simulink model "Prescan_Carsim_0118_repair_cs"  (R2019b)
settings: Solver=ode5  StartTime=0.0  StopTime=inf  FixedStep=1/1000  RelTol=1e-3
PreLoadFcn:
  | mbxruntime.callbacks.PreLoadFcn(bdroot);
PostLoadFcn:
  | mbxruntime.callbacks.PostLoadFcn(bdroot);
InitFcn:
  | mbxruntime.callbacks.InitFcn(bdroot);
  | Initialization_Func;
  | %T01_Init_2106;
StartFcn:
  | mbxruntime.callbacks.StartFcn(bdroot);
  | current_sys=gcs;
  | speedblock=Simulink.findBlocks(current_sys,'Name','speed_kmh_Gain');
  | h1=add_exec_event_listener(speedblock,'PostOutputs',@SpeedVisulization);
  | outblock=Simulink.findBlocks(current_sys,'Name','trajectorycurveoutput_Gain');
  | CurveTrajectoryListenerHandle=add_exec_event_listener(outblock,'PostOutputs',@TrajectoryCurve_CallBack);
  | lanedatablock=Simulink.findBlocks(current_sys,'Name','LaneData_Gain');
  | CurveLaneListenerHandle=add_exec_event_listener(lanedatablock,'PostOutputs',@CurveLane_CallBack);
StopFcn:
  | mbxruntime.callbacks.StopFcn(bdroot);
model workspace: external: MAT-File .\Prescan_Carsim_1230_cs_hws.mat (data not in the file)
undefined symbols (not defined in the file or in its folder): AAx, AAy, AAz, AVx, AVy, AVz, Ax, Ay, Az, canChannel, DiscIntNeverNeededParam, g, InitialDPMPDF_Comfort, InitialDPMPDF_Efficiency, InitialDPMPDF_Safety, InitialPDF_DEM, InitialPlanningParameter, Kf, Kr, Lr, M, mbxruntime, nG, NormalisedTrajectoryIndicator_Pool, Parameter_Indicator_LookUpTable, Prescan_Carsim_1230_cs_0658e9ca1334a8be, Prescan_Carsim_1230_cs_08c5eb9a1bd7376a, Prescan_Carsim_1230_cs_6cfd759b89b9fc85, Prescan_Carsim_1230_cs_9435cc1cceb5050d, Prescan_Carsim_1230_cs_ac716d34d49f74ab, Prescan_Carsim_1230_cs_be02757d7f212dd5, Rational_Coefficient_Learning, SteeringWheel, TrajectoryIndicatorRange, V, VehicleBaseLength, Vx, Vy, Vz, WheelL0, WheelL1, WheelR0, WheelR1
libraries: canmsglib x11, dsparch4 x6, canlib x3, PreScanSimulinkLibrary x3, Solver_SF x1, autolibshared x1
(part 1 of 8)
CloseFcn:
  | mbxruntime.callbacks.CloseFcn(bdroot);
settings Model: NumberOfSteps=100  Creator=PRESCAN  LastModifiedBy=CECLAB
settings DataIOCC: LimitDataPoints=on  SaveFormat=Array  SignalLoggingSaveFormat=ModelDataLogs  ReturnWorkspaceOutputs=off
settings OptimizationCC: DefaultParameterBehavior=Inlined  OptimizeBlockIOStorage=off  BufferReuse=off  GlobalBufferReuse=off  ExpressionFolding=off  ExpressionDepthLimit=2147483647  LocalBlockOutputs=off  InitFltsAndDblsToZero=on  LifeSpan=inf  OptimizeDataStoreBuffers=off  BusAssignmentInplaceUpdate=off
settings DebuggingCC: SaveWithParameterizedLinksMsg=none  UnderspecifiedInitializationDetection=Classic  MergeDetectMultiDrivingBlocksExec=none  SignalResolutionControl=TryResolveAllWithWarning  MultiTaskDSMMsg=warning  MultiTaskCondExecSysMsg=none  FcnCallInpInsideContextMsg=warning  StateNameClashWarn=warning  SFUnexpectedBacktrackingDiag=warning  SFNoUnconditionalDefaultTransitionDiag=warning  SFExecutionAtInitializationDiag=none  ArithmeticOperatorsInVariantConditions=warning
settings HardwareCC: ProdBitPerPointer=32  ProdBitPerSizeT=32  ProdBitPerPtrDiffT=32  ProdLargestAtomicFloat=None  ProdIntDivRoundTo=Undefined  ProdEndianess=Unspecified  ProdWordSize=32  ProdHWDeviceType=32-bit Generic
settings ModelReferenceCC: UpdateModelReferenceTargets=IfOutOfDate  PropagateSignalLabelsOutOfModel=off
settings SFSimCC: SimUseLocalCustomCode=off  SimParseCustomCode=off  CustomCodeUndefinedFunction=UseInterfaceOnly
settings SFSimCC: SimCustomHeaderCode=|
  | #include "prescan_alms_data.h"
  | #include "prescan.h"
  | #include "prescan_platform.h"
  | #include "prescan_aimsunturnindicatorsetter_data.h"
settings RTWCC: RTWUseLocalCustomCode=off
settings CodeAppCC: StateflowObjectComments=on
settings GRTTargetCC: TargetFcnLib=ansi_tfl_tmw.mat  TargetLangStandard=C89/C90 (ANSI)  GeneratePreprocessorConditionals=Disable all  CombineOutputUpdateFcns=off  GRTInterface=on
settings ConfigComp: CovMetricSettings=dw  CovHtmlReporting=on  CovSaveCumulativeToWorkspaceVar=on  CovSaveSingleToWorkspaceVar=on  CovExternalEMLEnable=off  CovSFcnEnable=off

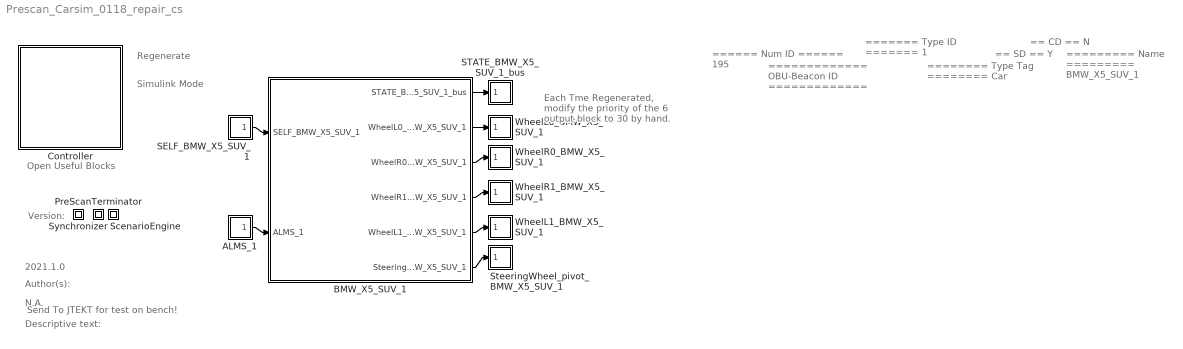
== system Prescan_Carsim_0118_repair_cs ==
  note: Each Tme Regenerated, modify the priority of the 6 output block to 30 by hand.
  note: Regenerate
  note: Simulink Mode
  note: Open Useful Blocks
  note: 2021.1.0
  note: Version:
  note: Author(s):
  note: N.A.
  note: Descriptive text:
  note: Send To JTEKT for test on bench!
  note: ======
      | Num ID
      | ======
      | 195
  note: =============
      | OBU-Beacon ID
      | =============
  note: =======
      | Type ID
      | =======
      | 1
  note: ========
      | Type Tag
      | ========
      | Car
  note: ==
      | SD
      | ==
      | Y
  note: ==
      | CD
      | ==
      | N
  note: =========
      | Name
      | =========
      | BMW_X5_SUV_1
  ALMS_1 : Subsystem  Tag=sensor/ALMS  Priority=30  LoadFcn=load('PrescanALMSData.mat');load('PrescanALMSMessage.mat');load('PrescanALMSPolynomial.mat')  mask(Analytical Lane Marker Sensor (ALMS) I/O){}
      mask help: The Analytical Lane Marker Sensor (ALMS) is a implementation of the Lane Marker Sensor, which provides information about the lane lines on the roads which are in view of the sensor.
      settings: OpenFcn=open_system([gcb '/Sensor'],'mask')
      mask Help: eval('openHelp(1466)')
      mask Display: image(imread('LaneMarkerSensorSL.png'))
  BMW_X5_SUV_1 : Subsystem  Tag=WorldObjectSubSystem  InitFcn=UniqueId = '1798';
      mask init:
      | modelPath = GenericModelHelper.getGenericModelFilePath('ModelDepo','Vehicles\BMW_X5\BMW_X5.pgmb','bfeb1c11467705ab888b3011684c848b');imagePath = GenericModelHelper.getCompilationPicture(modelPath, 'BMW_X5_HighPoly.png');
      mask Display: image(imread(imagePath));color('white');text(0, 0, ' ID=195\n')
  Controller : Subsystem  Description=8A3CD2955739A82C886C20AE3E253D78460D53180EE2C1B14CC08DF75A70BE77  Priority=-1  LoadFcn=load PreScanControllerData  mask(PreScan Simulation Controller){prescanversion='2021.1.0', ModelReferencing=off, TimeStep=50/1000, ControlMode=0, PreScanExecutionMode=on, ControllerCount=0, ControllerIndex=0, ControllerOptions=''}
      mask prompts: prescanversion "PreScan Version"; ModelReferencing "Use Model Referencing"; TimeStep "Upload Period [s]"; ControlMode "Control Mode"; PreScanExecutionMode "Execution Mode"; ControllerCount "Controller Count"; ControllerIndex "Controller Index"; ControllerOptions "Controller Options"
      mask help:
      | Please do not remove this block from the compilation sheet,
      | as it connects the model to the PreScan environment.
      mask init:
      | model = bdroot(gcb);
      | ExperimentFile = mbxruntime.findExperimentFile(model,true); %relative path
      | 
      | [d1, d2, d3, prescandata] = prescan_Settings();
      | ModelDepo = fullfile(prescandata,'ModelDepo'); 
      | 
      | RTmode = mbxruntime.getRTMode(model);
      | 
      | SimulationMode = get_param(bdroot,'SimulationMode');
      | if strcmp(SimulationMode, 'rapid-accelerator')
      |     SimulationMode = 'external';
      | end
      | TargetName = get_param(bdroot,'SystemTargetFile');
      settings: ModelCloseFcn=assignin('base',['model_closed_' bdroot],true);
      mask Help: eval('openHelp(812)')
      mask Display: image(imread('prescanlogo.ico'))
  PreScanTerminator : Subsystem  Tag=PreScanTerminator  Priority=999  LoadFcn=load PrescanTerminatorData  mask(PreScan Simulation Terminator){TimeStep=50/1000}
      mask prompts: TimeStep "Upload Period [s]"
      mask help:
      | Please do not remove this block from the compilation sheet as it
      | connects the model to the PreScan environment.
      mask Help: eval('openHelp(812)')
      mask Display: image(imread('prescanlogo.ico'))
  SELF_BMW_X5_SUV_1 : Subsystem  Tag=sensor/SelfPort  Priority=30  LoadFcn=load('PreScanSelfSensorData.mat')  mask(PreScan Source Block: SELF){}
      mask help:
      | The SELF port shows (state) information of the actor itself. The outputs are position in the experiment's axis system and the GPS coordinates, and the object's absolute velocity and compass heading.
      |
      | For more information, please click Help.
      settings: OpenFcn=open_system([gcb '/Sensor'],'mask')
      mask Help: eval('openHelp(462)')
      mask Display: image(imread('GPS.png'))
  STATE_BMW_X5_SUV_1_bus : Subsystem  Tag=actuator/StatePort  Priority=30  LoadFcn=load('PreScanStateActuatorData.mat')  mask(PreScan Sink Block: State){}
      mask help:
      | The Actor State contains a vector signal of size (9x1), containing the following signals:
      |
      | -  Position    	(x,y,z)             	[m]
      | -  Velocity    	(vx,vy,vz)         	[m/s]
      | -  Angles       	(Roll, Pitch, Yaw)	[rad]
      |
      | The Actor state is defined in the global axis system.
      | The state is superponed on the Initial position defined in the GUI.
      |
      | For more information, please click Help.
      settings: OpenFcn=open_system([gcb '/Actuator'],'mask')
      mask Help: eval('openHelp(222)')
      mask Display: image(imread('State.png'))
  ScenarioEngine : Subsystem  Tag=PreScanOpenScenarioBlock  Priority=0  LoadFcn=load PrescanSynchronizeData  mask(PreScan Simulation Core Block){TimeStep=50/1000}
      mask prompts: TimeStep "Timestep [s]"
      mask help:
      | Please do not remove this block from the PreScan compilation sheet,
      | as it contains essential configuration parameters for a PreScan simulation.
      settings: DeleteFcn=PreScanBlockDeleteFcn;
      mask Display: image(imread('prescanlogo.ico'))
  SteeringWheel_pivot_BMW_X5_SUV_1 : Subsystem  Tag=Actuator  Priority=30  LoadFcn=load('PrescanPoseData');load('PrescanXYZData');load('PreScanRPYData')
      mask help:
      | The VisuJoint block provides a way to adapt the location and orientation of a part of an object.
      |
      | For more information, please click Help.
      settings: OpenFcn=open_system([gcb '/Actuator'],'mask')
      mask Display: image(imread('Joint.png'))
  Synchronizer : Subsystem  Tag=PreScanSynchronizer  Priority=0  LoadFcn=load PrescanSynchronizeData  mask(PreScan Simulation Core Block){TimeStep=50/1000}
      mask prompts: TimeStep "Timestep [s]"
      mask help:
      | Please do not remove this block from the PreScan compilation sheet,
      | as it contains essential configuration parameters for a PreScan simulation.
      settings: DeleteFcn=PreScanBlockDeleteFcn;
      mask Display: image(imread('prescanlogo.ico'))
  WheelL0_BMW_X5_SUV_1 : Subsystem  Tag=Actuator  Priority=30  LoadFcn=load('PrescanPoseData');load('PrescanXYZData');load('PreScanRPYData')
      mask help:
      | The VisuJoint block provides a way to adapt the location and orientation of a part of an object.
      |
      | For more information, please click Help.
      settings: OpenFcn=open_system([gcb '/Actuator'],'mask')
      mask Display: image(imread('Joint.png'))
  WheelL1_BMW_X5_SUV_1 : Subsystem  Tag=Actuator  Priority=30  LoadFcn=load('PrescanPoseData');load('PrescanXYZData');load('PreScanRPYData')
      mask help:
      | The VisuJoint block provides a way to adapt the location and orientation of a part of an object.
      |
      | For more information, please click Help.
      settings: OpenFcn=open_system([gcb '/Actuator'],'mask')
      mask Display: image(imread('Joint.png'))
  WheelR0_BMW_X5_SUV_1 : Subsystem  Tag=Actuator  Priority=30  LoadFcn=load('PrescanPoseData');load('PrescanXYZData');load('PreScanRPYData')
      mask help:
      | The VisuJoint block provides a way to adapt the location and orientation of a part of an object.
      |
      | For more information, please click Help.
      settings: OpenFcn=open_system([gcb '/Actuator'],'mask')
      mask Display: image(imread('Joint.png'))
  WheelR1_BMW_X5_SUV_1 : Subsystem  Tag=Actuator  Priority=30  LoadFcn=load('PrescanPoseData');load('PrescanXYZData');load('PreScanRPYData')
      mask help:
      | The VisuJoint block provides a way to adapt the location and orientation of a part of an object.
      |
      | For more information, please click Help.
      settings: OpenFcn=open_system([gcb '/Actuator'],'mask')
      mask Display: image(imread('Joint.png'))
  wires:
  SELF_BMW_X5_SUV_1/1(SELF_BMW_X5_SUV_1) -> BMW_X5_SUV_1/1(SELF_BMW_X5_SUV_1)
  BMW_X5_SUV_1/1(STATE_BMW_X5_SUV_1_bus) -> STATE_BMW_X5_SUV_1_bus/1(STATE_BMW_X5_SUV_1_bus)
  ALMS_1/1(ALMS_1) -> BMW_X5_SUV_1/2(ALMS_1)
  BMW_X5_SUV_1/2(WheelL0_BMW_X5_SUV_1) -> WheelL0_BMW_X5_SUV_1/1(WheelL0_BMW_X5_SUV_1)
  BMW_X5_SUV_1/3(WheelR0_BMW_X5_SUV_1) -> WheelR0_BMW_X5_SUV_1/1(WheelR0_BMW_X5_SUV_1)
  BMW_X5_SUV_1/4(WheelR1_BMW_X5_SUV_1) -> WheelR1_BMW_X5_SUV_1/1(WheelR1_BMW_X5_SUV_1)
  BMW_X5_SUV_1/5(WheelL1_BMW_X5_SUV_1) -> WheelL1_BMW_X5_SUV_1/1(WheelL1_BMW_X5_SUV_1)
  BMW_X5_SUV_1/6(SteeringWheel_pivot_BMW_X5_SUV_1) -> SteeringWheel_pivot_BMW_X5_SUV_1/1(SteeringWheel_pivot_BMW_X5_SUV_1)

== system Prescan_Carsim_0118_repair_cs/ALMS_1 ==
  Sensor : S-Function  FunctionName=sfun_ALMS  Parameters=mbxruntime.parameters.convert(sensorID), mbxruntime.parameters.convert(detectableObjects), mbxruntime.parameters.convert(timestep)  SFunctionDeploymentMode=off  EnableBusSupport=off  mask(Analytical Lane Marker Sensor (ALMS) I/O){sensorID=15468, detectableObjects=30, timestep=1/20}
      mask prompts: sensorID "Sensor ID"; detectableObjects "Max detectable objects:"; timestep "MATLAB timestep:"
      mask help: The Analytical Lane Marker Sensor (ALMS) is a implementation of the Lane Marker Sensor, which provides information about the lane lines on the roads which are in view of the sensor.
      mask Help: eval('openHelp(1466)')
      mask Display: image(imread('LaneMarkerSensorSL.png'))
  ALMS_1 : Outport  Tag=outport/ALMS  OutDataTypeStr=Bus: PRESCAN_ALMS_MESSAGE  PortDimensions=30  SampleTime=1/20
  wires:
  Sensor/1 -> ALMS_1/1

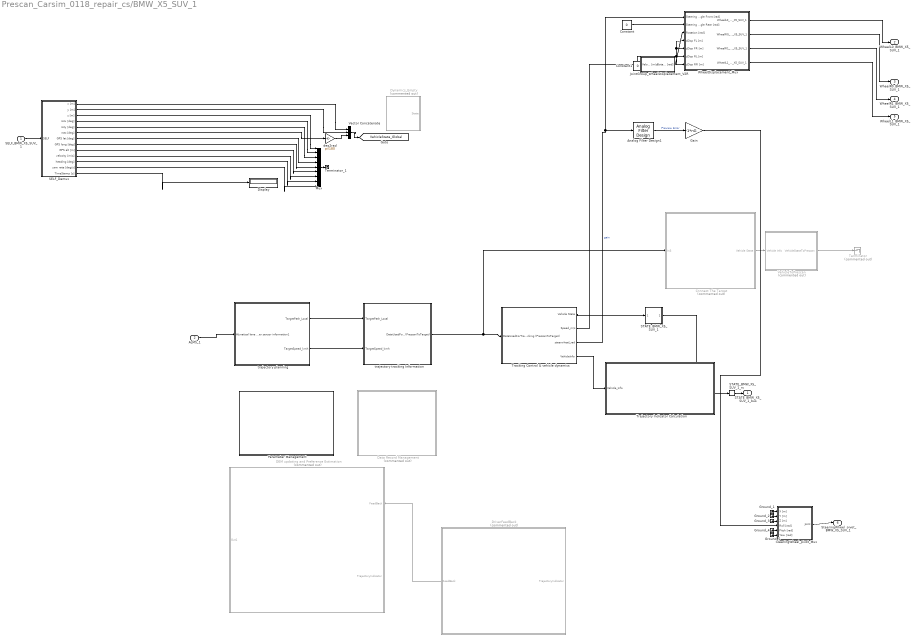
== system Prescan_Carsim_0118_repair_cs/BMW_X5_SUV_1 ==
  SELF_BMW_X5_SUV_1 : Inport  Tag=inport/SelfPort  OutDataTypeStr=Bus: PRESCAN_SELFSENSORDATA  PortDimensions=1  SampleTime=50/1000  BusOutputAsStruct=on
  ALMS_1 : Inport  Tag=inport/ALMS  Port=2  OutDataTypeStr=Bus: PRESCAN_ALMS_MESSAGE  PortDimensions=30  SampleTime=1/20  BusOutputAsStruct=on
  Analog Filter Design1 : dsparch4/Analog Filter Design  method=Butterworth  filttype=Lowpass  N=1  Wlo=1  Whi=80  Rp=2  Rs=40
  "Connect The Target " : Subsystem  Commented=on
  Constant : Constant  Value=0
  Constant1 : Constant  Value=0
  DEM updating and Preference Estimation : Subsystem  Commented=on
  Data Record Management : Subsystem  Commented=on
  Display : Display
  DriverFeedBack : Subsystem  Commented=on
  Dynamics_Empty : Subsystem  Tag=Dynamics_Empty  Commented=on
      mask Help: eval('openHelp(202)')
      mask Display: port_label('output', 1, 'State');text(0,0,' Empty\n')
  Gain : Gain  Gain=-1*nG
  Ground_{1..5} (5 alike) : Ground
  JointGroup_WheelDisplacement_V2R : Subsystem  Tag=mux/Wheels  mask(PreScan Velocity to Wheel Angle Block:){TimeStep=50/1000, TireRadius=0.29}
      mask prompts: TimeStep "Auto Assigned: Time Step [s]"; TireRadius "Tire Radius [m]"
      settings: DeleteFcn=PreScanBlockDeleteFcn;
      mask Display: disp('Velocity\nto\nWheelAngle')
  Mux : Mux  Inputs=9
  Parameter Management : Subsystem
  SELF_Demux : Subsystem  Tag=demux/SelfPort  mask(PreScan Demux Block:){}
      mask help:
      | The SELF port shows (state) information of the actor itself. The outputs are position in the experiment's axis system and the GPS coordinates, and the object's absolute velocity and compass heading.
      |
      | For more information, please click Help.
      settings: DeleteFcn=PreScanBlockDeleteFcn;
      mask Help: eval('openHelp(462)')
      mask Display:
      | port_label('output',1,'x [m]')
      | port_label('output',2,'y [m]')
      | port_label('output',3,'z [m]','texmode','on')
      | port_label('output',4,'Rotx [deg]','texmode','on')
      | port_label('output',5,'Roty [deg]','texmode','on')
      | port_label('output',6,'Rotz [deg]','texmode','on')
      | port_label('output',7,'GPS lat [deg]','texmode','on')
      | port_label('output',8,'GPS long [deg]','texmode','on')
      | port_label('output',9,'GPS alt [m]','texmode','on')
      | port_label('output',10,'Velocity [m/s]')
      | port_label('output',11,'Heading [deg]')
      | port_label('output',12,'Yaw rate [deg/s]')
      | port_label('output',13,'Timestamp [s]')
  STATE_BMW_X5_SUV_1 : Subsystem  Tag=mux/StatePort  Priority=0  LoadFcn=load PrescanStateActuatorData  mask(PreScan Sink Block: State){x0=0, y0=-1.75, z0=0.69, Roll0=0, Pitch0=0, Yaw0=0, TimeStep=1/20}
      mask prompts: x0 "Ini x-position VEHICLE wrt GLOBAL axis system [m]"; y0 "Ini y-position VEHICLE wrt GLOBAL axis system [m]"; z0 "Ini z-position VEHICLE wrt GLOBAL axis system [m]"; Roll0 "Ini roll-angle BODY wrt VEHICLE axis system [deg]"; Pitch0 "Ini pitch-angle BODY wrt VEHICLE axis system [deg]"; Yaw0 "Ini yaw-angle VEHICLE wrt GLOBAL axis system [deg]"; TimeStep "Auto-Assigned: Upload Period [s]"
      mask help:
      | The Actor State contains a vector signal of size (9x1), containing the following signals:
      |
      | -  Position                  (x,y,z)                                     [m]
      | -  Velocity                  (vx,vy,vz)                               [m/s]
      | -  Angles                    (Roll, Pitch, Yaw)                   [rad]
      |
      | The Actor state is defined in the global axis system.
      | The state is superponed on the Initial position defined in the GUI.
      |
      | For more information, please click Help.
      settings: DeleteFcn=PreScanBlockDeleteFcn;
      mask Help: eval('openHelp(222)')
      mask Display: image(imread('State.png'))
  STATE_BMW_X5_SUV_1_rc : RateTransition  Tag=mux_rc/StatePort  OutPortSampleTimeOpt=Inherit
  SteeringWheel_pivot_Mux : Subsystem  Tag=mux/Joint  mask(PreScan Mux Block){DisplayName=SteeringWheel}
      mask prompts: DisplayName "Display Name"
      mask help:
      | This block simulates a generic joint used for generic models. This joint can be enabled/disabled from the GUI.
      |
      | For more information, please click Help.
      settings: DeleteFcn=PreScanBlockDeleteFcn;
      mask Help: eval('openHelp(254)')
  Terminator : Terminator  Commented=on
  Terminator_1 : Terminator
  Tracking Control & vehicle dynamics : Subsystem
  Trajectory Indicator Calculation : Subsystem
  Vector Concatenate : Concatenate  NumInputs=3  Mode=Multidimensional array  ConcatenateDimension=2
  VehicleToPrescan : Subsystem  Commented=on
  WheelDisplacement_Mux : Subsystem  Tag=mux/JointGroup  mask(JointGroup){}
      mask help:
      | The JointGroup allows to control several Joints in one go, as defined for this particular model.
      | For more information, look in the PreScan manual in the section "Model Preparation Tool" -> "Joint Groups"
      |
      | For more information on the Joints simulink interface, press Help.
      mask Help: eval('openHelp(254)')
  deg2rad : Gain  Gain=pi/180
  trajectory planning : Subsystem
  trajectory tracking Information : Subsystem
  STATE_BMW_X5_SUV_1_bus : Outport  Tag=outport/StatePort  OutDataTypeStr=Bus: PRESCAN_STATEACTUATORDATA  PortDimensions=1  SampleTime=50/1000
  WheelL0_BMW_X5_SUV_1 : Outport  Tag=outport/JointActuator  Port=2  OutDataTypeStr=Bus: PRESCAN_POSE_DATA  SampleTime=50/1000
  WheelR0_BMW_X5_SUV_1 : Outport  Tag=outport/JointActuator  Port=3  OutDataTypeStr=Bus: PRESCAN_POSE_DATA  SampleTime=50/1000
  WheelR1_BMW_X5_SUV_1 : Outport  Tag=outport/JointActuator  Port=4  OutDataTypeStr=Bus: PRESCAN_POSE_DATA  SampleTime=50/1000
  WheelL1_BMW_X5_SUV_1 : Outport  Tag=outport/JointActuator  Port=5  OutDataTypeStr=Bus: PRESCAN_POSE_DATA  SampleTime=50/1000
  SteeringWheel_pivot_BMW_X5_SUV_1 : Outport  Tag=outport/JointActuator  Port=6  OutDataTypeStr=Bus: PRESCAN_POSE_DATA  SampleTime=50/1000
  tag scope: VehicleState_Global=global
  wires:
  Vector Concatenate/1 -> [VehicleState_Global]
  SELF_Demux/1(x [m]) -> Vector Concatenate/1
  SELF_Demux/2(y [m]) -> Vector Concatenate/2
  SELF_Demux/6(rotz [deg]) -> deg2rad/1
  SELF_Demux/3(z [m]) -> Mux/1
  SELF_Demux/4(rotx [deg]) -> Mux/2
  SELF_Demux/5(roty [deg]) -> Mux/3
  SELF_Demux/7(GPS lat [deg]) -> Mux/4
  SELF_Demux/8(GPS long [deg]) -> Mux/5
  SELF_Demux/9(GPS alt [m]) -> Mux/6
  SELF_Demux/10(velocity [m/s]) -> Mux/7
  SELF_Demux/11(heading [deg]) -> Mux/8
  SELF_Demux/12(yaw rate [deg/s]) -> Mux/9
  STATE_BMW_X5_SUV_1/1(StateBus) -> STATE_BMW_X5_SUV_1_rc/1
  trajectory planning/1(TargetPath_Local) -> trajectory tracking Information/1(TargetPath_Local)
  trajectory tracking Information/1(DataUsedForTracking (PrescanToTarget)) -> "Connect The Target "/1(In3), Tracking Control & vehicle dynamics/1(DataUsedForTracking (PrescanToTarget))
  trajectory planning/2(TargetSpeed_kmh) -> trajectory tracking Information/2(TargetSpeed_kmh)
  SELF_BMW_X5_SUV_1/1 -> SELF_Demux/1(SELF)
  STATE_BMW_X5_SUV_1_rc/1 -> STATE_BMW_X5_SUV_1_bus/1
  "Connect The Target "/1(Vehicle State) -> VehicleToPrescan/1(Vehicle Info)
  ALMS_1/1 -> trajectory planning/1(Alynatical lane marker sensor information1)
  Tracking Control & vehicle dynamics/3("steerwheel_rad ") -> WheelDisplacement_Mux/1(Steering Angle Front [rad]), Analog Filter Design1/1  "gain"
  Gain/1 -> SteeringWheel_pivot_Mux/4(Roll [rad])
  DriverFeedBack/1(FeedBack) -> DEM updating and Preference Estimation/1(FeedBack)
  Tracking Control & vehicle dynamics/1(Vehicle State) -> STATE_BMW_X5_SUV_1/1(State)
  Tracking Control & vehicle dynamics/4(VehicleInfo) -> Trajectory Indicator Calculation/1(Vehicle_Info)
  SELF_Demux/13(TimeStamp [s]) -> Display/1
  VehicleToPrescan/1(VehicleStateToPrescan) -> Terminator/1
  deg2rad/1 -> Vector Concatenate/3
  Tracking Control & vehicle dynamics/2(Speed_m/s) -> JointGroup_WheelDisplacement_V2R/1(Velocity [m/s])
  Constant/1 -> WheelDisplacement_Mux/2(Steering Angle Rear [rad])
  Constant1/1 -> WheelDisplacement_Mux/7(zDisp RR [m]), WheelDisplacement_Mux/6(zDisp RL [m]), WheelDisplacement_Mux/5(zDisp FR [m]), WheelDisplacement_Mux/4(zDisp FL [m])
  Analog Filter Design1/1 -> Gain/1  "Preview Error"
  WheelDisplacement_Mux/1(WheelL0_BMW_X5_SUV_1) -> WheelL0_BMW_X5_SUV_1/1
  WheelDisplacement_Mux/2(WheelR0_BMW_X5_SUV_1) -> WheelR0_BMW_X5_SUV_1/1
  WheelDisplacement_Mux/3(WheelR1_BMW_X5_SUV_1) -> WheelR1_BMW_X5_SUV_1/1
  WheelDisplacement_Mux/4(WheelL1_BMW_X5_SUV_1) -> WheelL1_BMW_X5_SUV_1/1
  JointGroup_WheelDisplacement_V2R/1(Rotation [rad]) -> WheelDisplacement_Mux/3(Rotation [rad])
  SteeringWheel_pivot_Mux/1(Joint) -> SteeringWheel_pivot_BMW_X5_SUV_1/1
  Mux/1 -> Terminator_1/1
  Ground_1/1 -> SteeringWheel_pivot_Mux/1(X [m])
  Ground_2/1 -> SteeringWheel_pivot_Mux/2(Y [m])
  Ground_3/1 -> SteeringWheel_pivot_Mux/3(Z [m])
  Ground_4/1 -> SteeringWheel_pivot_Mux/5(Pitch [rad])
  Ground_5/1 -> SteeringWheel_pivot_Mux/6(Yaw [rad])

== system Prescan_Carsim_0118_repair_cs/Controller ==
  Terminator : Terminator
  sfun_Controller : S-Function  FunctionName=sfun_Controller  Parameters=SParameter1, SParameter2, SParameter3, SParameter4, SParameter5, SParameter6, SParameter7, SParameter8, SParameter9, SParameter10, SampleTime  SFunctionDeploymentMode=off  EnableBusSupport=off  mask(Legacy Function){SFunctionSpec=void prescan_outputFcn(void** work1, PRESCAN_CONTROLLERDATA y1[1]), SParameter1=uint8([ExperimentFile 0]), SParameter2=uint8([ModelDepo 0]), SParameter3=uint8([ControllerOptions 0]), SParameter4=RTmode, SParameter5=PreScanExecutionMode, SParameter6=ControlMode, SParameter7=ControllerCount, SParameter8=ControllerIndex, SParameter9=uint8([SimulationMode 0]), SParameter10=uint8([TargetName 0]), SampleTime=TimeStep, ShowSpec=on}
      mask prompts: SParameter1 "P1:"; SParameter2 "P2:"; SParameter3 "P3:"; SParameter4 "P4:"; SParameter5 "P5:"; SParameter6 "P6:"; SParameter7 "P7:"; SParameter8 "P8:"; SParameter9 "P9:"; SParameter10 "P10:"; SampleTime "Sample time (-1 for inherited):"; ShowSpec "Display function specification"
      mask help:
      | This block allows you to call the legacy functions specified by the following Legacy Code Tool definition:
      | def.SFunctionName = 'sfun_Controller';
      | def.OutputFcnSpec = 'void prescan_outputFcn(void** work1, PRESCAN_CONTROLLERDATA y1[1])';
      | def.StartFcnSpec = 'void prescan_startFcn(void ** work1, uint8 p1[], uint8 p2[], uint8 p3[], double p4, double p5, double p6, double p7, double p8, uint8 p9[], uint8 p10[])';
      | def.TerminateFcnSpec = 'void prescan_terminateFcn(void** work1)';
      | def.HeaderFiles = {'prescan_controller_data.h', 'prescan_SFunLibrary.h', 'prescan_CreateLogHandler.h', 'prescan_CreateErrorHandler.h', 'prescan_modify.h', 'ModuleDLL.h'};
      | def.SourceFiles = {'prescan_MexLogHandler.c', 'prescan_SimStructErrorHandler.c', 'prescan_LogHandler.c', 'prescan_ErrorHandler.c', 'prescan_Modify.c'};
      | def.HostLibFiles = {'sensorinterfaced.lib'};
      | def.TargetLibFiles = {'sensorinterfaced.so'};
      | def.IncPaths = {'.', 'C:\projects\prescan\rt_vislibrary\vis\..\pimp\include\sensors\InterfaceRTW'};
      | def.SrcPaths = {'C:\projects\prescan\rt_vislibrary\vis\..\pimp\include\sensors\InterfaceRTW', 'C:\projects\prescan\rt_vislibrary\vis\..\pimp\include\sensors\InterfaceRTW\ccurrt'};
      | def.LibPaths = {'C:\\projects\\prescan\\vislibrary_build\lib'};
      | def.SampleTime = 'parameterized';
      mask Help: <p>This block was generated automatically by the Legacy Code Tool. For detailed help on this tool, call<a href="matlab:legacy_code('help')"> legacy_code('help')</a>.</p>
      mask Callback ShowSpec:
      | if strcmp(get_param(gcbh, 'ShowSpec'), 'on')
      |   set_param(gcbh, 'MaskDisplay', sprintf('fprintf(''%s'');', get_param(gcbh, 'SFunctionSpec')));
      | else
      |   set_param(gcbh, 'MaskDisplay', sprintf('fprintf(''%s'');', get_param(gcbh, 'FunctionName')));
      | end
      mask Display: fprintf('void prescan_outputFcn(void** work1, PRESCAN_CONTROLLERDATA y1[1])');
  wires:
  sfun_Controller/1 -> Terminator/1

== system Prescan_Carsim_0118_repair_cs/PreScanTerminator ==
  Terminator : Terminator
  sfun_Terminator : S-Function  FunctionName=sfun_Terminator  Parameters=SampleTime  SFunctionDeploymentMode=off  EnableBusSupport=off  mask(Legacy Function){SFunctionSpec=void prescan_terminator_outputFcn(void ** work1, PRESCAN_TERMINATORDATA y1[1]), SampleTime=TimeStep, ShowSpec=on}
      mask prompts: SampleTime "Sample time (-1 for inherited):"; ShowSpec "Display function specification"
      mask help:
      | This block allows you to call the legacy functions specified by the following Legacy Code Tool definition:
      | def.SFunctionName = 'sfun_Terminator';
      | def.OutputFcnSpec = 'void prescan_terminator_outputFcn(void ** work1, PRESCAN_TERMINATORDATA y1[1])';
      | def.StartFcnSpec = 'void prescan_terminator_startFcn(void ** work1)';
      | def.TerminateFcnSpec = 'void prescan_terminator_terminateFcn(void ** work1)';
      | def.HeaderFiles = {'prescan_terminator_data.h'};
      | def.HostLibFiles = {'sensorinterfaced.lib'};
      | def.IncPaths = {'src', 'C:\prescandev\vislibrary\vis\..\pimp\include\sensors\InterfaceRTW'};
      | def.SrcPaths = {'src'};
      | def.LibPaths = {'C:\\prescandev\\vislibrary_build\lib'};
      | def.SampleTime = 'parameterized';
      | def.Options.language = 'C';
      mask Help: <p>This block was generated automatically by the Legacy Code Tool. For detailed help on this tool, call<a href="matlab:legacy_code('help')"> legacy_code('help')</a>.</p>
      mask Callback ShowSpec:
      | if strcmp(get_param(gcbh, 'ShowSpec'), 'on')
      |   set_param(gcbh, 'MaskDisplay', sprintf('fprintf(''%s'');', get_param(gcbh, 'SFunctionSpec')));
      | else
      |   set_param(gcbh, 'MaskDisplay', sprintf('fprintf(''%s'');', get_param(gcbh, 'FunctionName')));
      | end
      mask Display: fprintf('void prescan_terminator_outputFcn(void ** work1, PRESCAN_TERMINATORDATA y1[1])');
  wires:
  sfun_Terminator/1 -> Terminator/1

== system Prescan_Carsim_0118_repair_cs/SELF_BMW_X5_SUV_1 ==
  Sensor : S-Function  FunctionName=sfun_SelfSensor  Parameters=mbxruntime.parameters.convert(UniqueID), mbxruntime.parameters.convert(TimeStep)  SFunctionDeploymentMode=off  EnableBusSupport=off  mask(PreScan Source Block: SELF){UniqueID=1798, TimeStep=50/1000}
      mask prompts: UniqueID "Auto-Assigned: Unique ID"; TimeStep "Auto-Assigned: Upload Period [s]"
      mask help:
      | The SELF port shows (state) information of the actor itself. The outputs are position in the experiment's axis system and the GPS coordinates, and the object's absolute velocity and compass heading.
      |
      | For more information, please click Help.
      mask Help: eval('openHelp(462)')
      mask Display: image(imread('GPS.png'))
  SELF_BMW_X5_SUV_1 : Outport  Tag=outport/SelfPort  OutDataTypeStr=Bus: PRESCAN_SELFSENSORDATA  PortDimensions=1  SampleTime=50/1000
  wires:
  Sensor/1 -> SELF_BMW_X5_SUV_1/1

== system Prescan_Carsim_0118_repair_cs/STATE_BMW_X5_SUV_1_bus ==
  STATE_BMW_X5_SUV_1_bus : Inport  Tag=inport/StatePort  OutDataTypeStr=Bus: PRESCAN_STATEACTUATORDATA  PortDimensions=1  SampleTime=50/1000  BusOutputAsStruct=on
  Actuator : S-Function  FunctionName=sfun_StateActuator  Parameters=mbxruntime.parameters.convert(UniqueID), mbxruntime.parameters.convert(TimeStep)  SFunctionDeploymentMode=off  EnableBusSupport=off  mask(PreScan Sink Block: State){UniqueID=1798, TimeStep=50/1000}
      mask prompts: UniqueID "Auto-Assigned: Unique ID"; TimeStep "Auto-Assigned: Upload Period [s]"
      mask help:
      | The Actor State contains a vector signal of size (9x1), containing the following signals:
      |
      | -  Position    	(x,y,z)             	[m]
      | -  Velocity    	(vx,vy,vz)         	[m/s]
      | -  Angles       	(Roll, Pitch, Yaw)	[rad]
      |
      | The Actor state is defined in the global axis system.
      | The state is superponed on the Initial position defined in the GUI.
      |
      | For more information, please click Help.
      mask Help: eval('openHelp(222)')
      mask Display: image(imread('State.png'))
  wires:
  STATE_BMW_X5_SUV_1_bus/1 -> Actuator/1

== system Prescan_Carsim_0118_repair_cs/ScenarioEngine ==
  Clock1 : Clock
  Stop Simulation : Stop
  sfun_ScenarioEngine1 : S-Function  FunctionName=sfun_ScenarioEngine  Parameters=TimeStep  SFunctionDeploymentMode=off  EnableBusSupport=off
  wires:
  sfun_ScenarioEngine1/1 -> Stop Simulation/1
  Clock1/1 -> sfun_ScenarioEngine1/1

== system Prescan_Carsim_0118_repair_cs/SteeringWheel_pivot_BMW_X5_SUV_1 ==
  SteeringWheel_pivot_BMW_X5_SUV_1 : Inport  Tag=inport/JointActuator  OutDataTypeStr=Bus: PRESCAN_POSE_DATA  SampleTime=50/1000  BusOutputAsStruct=on
  Actuator : Subsystem  Tag=VisuJoint  mask(PreScan Sink Block: VisuJoint){UniqueID=1798, Translate_ObjectID3D=BMW_X5_SUV_1.SteeringWheel_pivot, Rotate_ObjectID3D=BMW_X5_SUV_1.SteeringWheel_pivot, TimeStep=50/1000, DisplayName=[]}
      mask prompts: UniqueID "Parent Unique ID"; Translate_ObjectID3D "Translate Object Name"; Rotate_ObjectID3D "Rotate Object Name"; TimeStep "Simulation Step"; DisplayName "Display Name"
      mask help:
      | The VisuJoint block provides a way to adapt the location and orientation of a part of an object.
      |
      | For more information, please click Help.
      settings: DeleteFcn=PreScanBlockDeleteFcn;
      mask Help: eval('openHelp(223)')
      mask Display: image(imread('Joint.png'))
  wires:
  SteeringWheel_pivot_BMW_X5_SUV_1/1 -> Actuator/1(Joint)

== system Prescan_Carsim_0118_repair_cs/Synchronizer ==
  Bus Selector1 : BusSelector  OutputSignals=FederateStopped
  Stop Simulation : Stop
  sfun_Synchronizer : S-Function  FunctionName=sfun_Synchronizer  Parameters=SampleTime  SFunctionDeploymentMode=off  EnableBusSupport=off  mask(Legacy Function){SFunctionSpec=void prescan_synchronizer_outputFcn(void ** work1, PRESCAN_SYNCHRONIZEDATA y1[1]), SampleTime=TimeStep, ShowSpec=on}
      mask prompts: SampleTime "Sample time (-1 for inherited):"; ShowSpec "Display function specification"
      mask help:
      | This block allows you to call the legacy functions specified by the following Legacy Code Tool definition:
      | def.SFunctionName = 'sfun_Synchronizer';
      | def.OutputFcnSpec = 'void prescan_synchronizer_outputFcn(void ** work1, PRESCAN_TIMESTAMPDATA u1[1], PRESCAN_SYNCHRONIZEDATA y1[1])';
      | def.StartFcnSpec = 'void prescan_synchronizer_startFcn(void ** work1)';
      | def.TerminateFcnSpec = 'void prescan_synchronizer_terminateFcn(void ** work1)';
      | def.HeaderFiles = {'prescan_synchronizer_data.h'};
      | def.HostLibFiles = {'sensorinterfaced.lib'};
      | def.IncPaths = {'src', 'C:\prescandev\vislibrary\vis\..\pimp\include\sensors\InterfaceRTW'};
      | def.SrcPaths = {'src'};
      | def.LibPaths = {'C:\\prescandev\\vislibrary_build\lib'};
      | def.SampleTime = 'parameterized';
      | def.Options.language = 'C';
      mask Help: <p>This block was generated automatically by the Legacy Code Tool. For detailed help on this tool, call<a href="matlab:legacy_code('help')"> legacy_code('help')</a>.</p>
      mask Callback ShowSpec:
      | if strcmp(get_param(gcbh, 'ShowSpec'), 'on')
      |   set_param(gcbh, 'MaskDisplay', sprintf('fprintf(''%s'');', get_param(gcbh, 'SFunctionSpec')));
      | else
      |   set_param(gcbh, 'MaskDisplay', sprintf('fprintf(''%s'');', get_param(gcbh, 'FunctionName')));
      | end
      mask Display: fprintf('void prescan_synchronizer_outputFcn(void ** work1, PRESCAN_SYNCHRONIZEDATA y1[1])');
  wires:
  sfun_Synchronizer/1 -> Bus Selector1/1
  Bus Selector1/1 -> Stop Simulation/1  "<FederateStopped>"

== system Prescan_Carsim_0118_repair_cs/WheelL0_BMW_X5_SUV_1 ==
  WheelL0_BMW_X5_SUV_1 : Inport  Tag=inport/JointActuator  OutDataTypeStr=Bus: PRESCAN_POSE_DATA  SampleTime=50/1000  BusOutputAsStruct=on
  Actuator : Subsystem  Tag=VisuJoint  mask(PreScan Sink Block: VisuJoint){UniqueID=1798, Translate_ObjectID3D=BMW_X5_SUV_1.WheelL0, Rotate_ObjectID3D=BMW_X5_SUV_1.WheelL0, TimeStep=50/1000, DisplayName=[]}
      mask prompts: UniqueID "Parent Unique ID"; Translate_ObjectID3D "Translate Object Name"; Rotate_ObjectID3D "Rotate Object Name"; TimeStep "Simulation Step"; DisplayName "Display Name"
      mask help:
      | The VisuJoint block provides a way to adapt the location and orientation of a part of an object.
      |
      | For more information, please click Help.
      settings: DeleteFcn=PreScanBlockDeleteFcn;
      mask Help: eval('openHelp(223)')
      mask Display: image(imread('Joint.png'))
  wires:
  WheelL0_BMW_X5_SUV_1/1 -> Actuator/1(Joint)

== system Prescan_Carsim_0118_repair_cs/WheelL1_BMW_X5_SUV_1 ==
  WheelL1_BMW_X5_SUV_1 : Inport  Tag=inport/JointActuator  OutDataTypeStr=Bus: PRESCAN_POSE_DATA  SampleTime=50/1000  BusOutputAsStruct=on
  Actuator : Subsystem  Tag=VisuJoint  mask(PreScan Sink Block: VisuJoint){UniqueID=1798, Translate_ObjectID3D=BMW_X5_SUV_1.WheelL1, Rotate_ObjectID3D=BMW_X5_SUV_1.WheelL1, TimeStep=50/1000, DisplayName=[]}
      mask prompts: UniqueID "Parent Unique ID"; Translate_ObjectID3D "Translate Object Name"; Rotate_ObjectID3D "Rotate Object Name"; TimeStep "Simulation Step"; DisplayName "Display Name"
      mask help:
      | The VisuJoint block provides a way to adapt the location and orientation of a part of an object.
      |
      | For more information, please click Help.
      settings: DeleteFcn=PreScanBlockDeleteFcn;
      mask Help: eval('openHelp(223)')
      mask Display: image(imread('Joint.png'))
  wires:
  WheelL1_BMW_X5_SUV_1/1 -> Actuator/1(Joint)

== system Prescan_Carsim_0118_repair_cs/WheelR0_BMW_X5_SUV_1 ==
  WheelR0_BMW_X5_SUV_1 : Inport  Tag=inport/JointActuator  OutDataTypeStr=Bus: PRESCAN_POSE_DATA  SampleTime=50/1000  BusOutputAsStruct=on
  Actuator : Subsystem  Tag=VisuJoint  mask(PreScan Sink Block: VisuJoint){UniqueID=1798, Translate_ObjectID3D=BMW_X5_SUV_1.WheelR0, Rotate_ObjectID3D=BMW_X5_SUV_1.WheelR0, TimeStep=50/1000, DisplayName=[]}
      mask prompts: UniqueID "Parent Unique ID"; Translate_ObjectID3D "Translate Object Name"; Rotate_ObjectID3D "Rotate Object Name"; TimeStep "Simulation Step"; DisplayName "Display Name"
      mask help:
      | The VisuJoint block provides a way to adapt the location and orientation of a part of an object.
      |
      | For more information, please click Help.
      settings: DeleteFcn=PreScanBlockDeleteFcn;
      mask Help: eval('openHelp(223)')
      mask Display: image(imread('Joint.png'))
  wires:
  WheelR0_BMW_X5_SUV_1/1 -> Actuator/1(Joint)

== system Prescan_Carsim_0118_repair_cs/WheelR1_BMW_X5_SUV_1 ==
  WheelR1_BMW_X5_SUV_1 : Inport  Tag=inport/JointActuator  OutDataTypeStr=Bus: PRESCAN_POSE_DATA  SampleTime=50/1000  BusOutputAsStruct=on
  Actuator : Subsystem  Tag=VisuJoint  mask(PreScan Sink Block: VisuJoint){UniqueID=1798, Translate_ObjectID3D=BMW_X5_SUV_1.WheelR1, Rotate_ObjectID3D=BMW_X5_SUV_1.WheelR1, TimeStep=50/1000, DisplayName=[]}
      mask prompts: UniqueID "Parent Unique ID"; Translate_ObjectID3D "Translate Object Name"; Rotate_ObjectID3D "Rotate Object Name"; TimeStep "Simulation Step"; DisplayName "Display Name"
      mask help:
      | The VisuJoint block provides a way to adapt the location and orientation of a part of an object.
      |
      | For more information, please click Help.
      settings: DeleteFcn=PreScanBlockDeleteFcn;
      mask Help: eval('openHelp(223)')
      mask Display: image(imread('Joint.png'))
  wires:
  WheelR1_BMW_X5_SUV_1/1 -> Actuator/1(Joint)

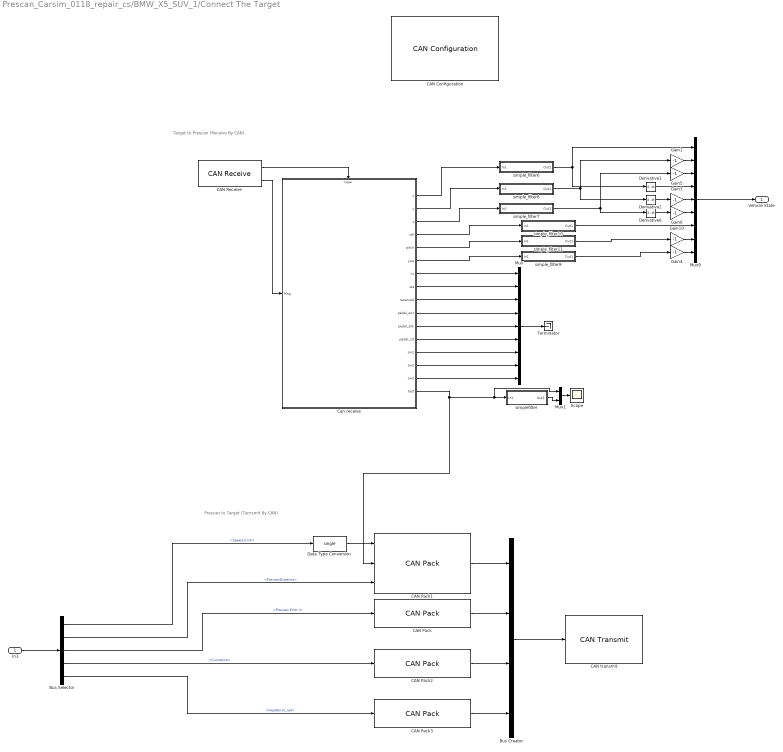
== system Prescan_Carsim_0118_repair_cs/BMW_X5_SUV_1/Connect The Target  ==
  note: Target to Prescan (Receive By CAN)
  note: Prescan to Target (Tarnsmit By CAN)
  In3 : Inport
  Bus Creator : BusCreator  Inputs=4
  Bus Selector : BusSelector  OutputSignals=Speed_Kmh,PreviewDistance,Preview Error I,Curvature,HeadError_rad
  CAN Configuration : canlib/CAN Configuration  BlockHandle=14.0012  Device=Kvaser USBcan II 1 (Channel 1)  DeviceMenu=Kvaser USBcan II 1 (Channel 1)  ObjConstructor=canChannel('Kvaser', 'USBcan II 1', 1)  BusSpeed=1000000  EnableBitParameters=off  SJW=1  TSEG1=4  TSEG2=3  NSamples=1  AckMode=Normal
      settings: SourceProductName=Vehicle Network Toolbox  SourceProductBaseCode=VN
  CAN Pack : canmsglib/CAN Pack  MsgList=(none)  MsgName=VSS1  MsgIDType=Standard (11-bit identifier)  MsgIdentifier=501  MsgLength=8  Remote=off  ApplyMinMax=off  BusOutput=off  SignalInfo={ 'previewError', '0', '64', 'LE', 'double', 'Standard', '0', '1', '0', '-Inf', 'Inf' }
      settings: SourceProductName=Simulink Real-Time  SourceProductBaseCode=XP  DataFormat=manually specified signals
  CAN Pack1 : canmsglib/CAN Pack  MsgList=(none)  MsgName=CAN Msg  MsgIDType=Standard (11-bit identifier)  MsgIdentifier=500  MsgLength=8  Remote=off  ApplyMinMax=off  BusOutput=off  SignalInfo={ 'Vx_des', '16', '32', 'LE', 'single', 'Standard', '0', '1', '0', '-Inf', 'Inf'; 'detection', '48', '16', 'LE', 'unsigned', 'Standard', '0', '1', '0', '-Inf', 'Inf'; 'previewDistance', '0', '16', 'LE', 'unsigned', 'Standard', '0', '1', '0', '-Inf', 'Inf' }
      settings: SourceProductName=Vehicle Network Toolbox  SourceProductBaseCode=VN  DataFormat=manually specified signals
  CAN Pack2 : canmsglib/CAN Pack  MsgList=(none)  MsgName=VSS2  MsgIDType=Standard (11-bit identifier)  MsgIdentifier=502  MsgLength=8  Remote=off  ApplyMinMax=off  BusOutput=off  SignalInfo={ 'curvature', '0', '64', 'LE', 'double', 'Standard', '0', '1', '0', '-Inf', 'Inf' }
      settings: SourceProductName=Simulink Real-Time  SourceProductBaseCode=XP  DataFormat=manually specified signals
  CAN Pack3 : canmsglib/CAN Pack  MsgList=(none)  MsgName=VSS1  MsgIDType=Standard (11-bit identifier)  MsgIdentifier=503  MsgLength=8  Remote=off  ApplyMinMax=off  BusOutput=off  SignalInfo={ 'head_error', '0', '64', 'LE', 'double', 'Standard', '0', '1', '0', '-Inf', 'Inf' }
      settings: SourceProductName=Simulink Real-Time  SourceProductBaseCode=XP  DataFormat=manually specified signals
  CAN Receive : canlib/CAN Receive  BlockHandle=19.0012  Device=Kvaser USBcan II 1 (Channel 1)  DeviceMenu=Kvaser USBcan II 1 (Channel 1)  ObjConstructor=canChannel('Kvaser', 'USBcan II 1', 1)  EnableStandardIDsFilter=off  StdIDsCombo=Allow all  StandardIDs=0  EnableExtendedIDsFilter=off  ExtIDsCombo=Allow all  ExtendedIDs=0  SampleTime=-1  MsgsPerTimestep=all  InternalFilterUpdateStatus=on  BusOutput=on
      settings: SourceProductName=Vehicle Network Toolbox  SourceProductBaseCode=VN
  CAN transmit : canlib/CAN Transmit  BlockHandle=20.0012  Device=Kvaser USBcan II 1 (Channel 1)  DeviceMenu=Kvaser USBcan II 1 (Channel 1)  ObjConstructor=canChannel('Kvaser', 'USBcan II 1', 1)  EnablePeriodicTransmit=off  MessagePeriod=1.000
      settings: SourceProductName=Vehicle Network Toolbox  SourceProductBaseCode=VN
  Can receive : Subsystem  TreatAsAtomicUnit=on
  Data Type Conversion : DataTypeConversion  OutDataTypeStr=single
  Derivative1 : Derivative
  Derivative2 : Derivative
  Derivative6 : Derivative
  Gain{1,3..6,10} (6 alike) : Gain  Gain=-1
  Mux : Mux  Inputs=9
  Mux1 : Mux  Inputs=2
  Mux9 : Mux  Inputs=9
  Scope : Scope
  Terminator : Terminator
  simple_filter10 : Subsystem
  simple_filter11 : Subsystem
  simple_filter6 : Subsystem
  simple_filter7 : Subsystem
  simple_filter8 : Subsystem
  simple_filter9 : Subsystem
  simplefilter : Subsystem
  Vehicle State : Outport
  wires:
  Mux9/1 -> Vehicle State/1
  Bus Selector/5 -> CAN Pack3/1  "<HeadError_rad>"
  Bus Selector/4 -> CAN Pack2/1  "<Curvature>"
  In3/1 -> Bus Selector/1
  CAN Pack1/1 -> Bus Creator/1
  Bus Selector/1 -> Data Type Conversion/1  "<Speed_Kmh>"
  Data Type Conversion/1 -> CAN Pack1/1
  Bus Selector/3 -> CAN Pack/1  "<Preview Error I>"
  CAN Pack/1 -> Bus Creator/2
  CAN Pack2/1 -> Bus Creator/3
  CAN Pack3/1 -> Bus Creator/4
  Bus Creator/1 -> CAN transmit/1
  Bus Selector/2 -> CAN Pack1/3  "<PreviewDistance>"
  CAN Receive/2 -> Can receive/1(Msg)
  CAN Receive/1 -> Can receive/Trigger
  Derivative6/1 -> Gain6/1
  Derivative2/1 -> Gain3/1
  Gain6/1 -> Mux9/6
  simple_filter6/1(Out1) -> Derivative1/1, Mux9/1
  simple_filter7/1(Out1) -> Derivative6/1, Gain5/1
  Gain1/1 -> Mux9/2
  Can receive/2(y) -> simple_filter8/1(In1)
  Can receive/3(z) -> simple_filter7/1(In1)
  Can receive/6(yaw) -> simple_filter9/1(In1)
  Gain5/1 -> Mux9/3
  Gain4/1 -> Mux9/9
  Gain3/1 -> Mux9/5
  simple_filter8/1(Out1) -> Gain1/1, Derivative2/1
  Can receive/5(pitch) -> simple_filter11/1(In1)
  simple_filter11/1(Out1) -> Gain10/1
  Can receive/1(x) -> simple_filter6/1(In1)
  Derivative1/1 -> Mux9/4
  simple_filter9/1(Out1) -> Gain4/1
  Gain10/1 -> Mux9/8
  Can receive/4(roll) -> simple_filter10/1(In1)
  Can receive/7(vx) -> Mux/1
  Can receive/8(sta) -> Mux/2
  Can receive/9(reserved) -> Mux/3
  Can receive/10(pedal_acc) -> Mux/4
  Can receive/11(pedal_brk) -> Mux/5
  Can receive/12(pedal_clt) -> Mux/6
  Can receive/13(sw1) -> Mux/7
  Can receive/14(sw2) -> Mux/8
  Can receive/15(sw3) -> Mux/9
  Mux/1 -> Terminator/1
  simplefilter/1(Out1) -> Mux1/2
  Can receive/16(test) -> Mux1/1, simplefilter/1(In1), CAN Pack1/2
  Mux1/1 -> Scope/1
  simple_filter10/1(Out1) -> Mux9/7

== system Prescan_Carsim_0118_repair_cs/BMW_X5_SUV_1/DEM updating and Preference Estimation ==
  FeedBack : Inport
      settings: AttributesFormatString=|
      | 0: There is no comparison
      | 1: Prefer the former one
      | 2：Prefer the latter one
      | 3: No obvious preference
  TrajectoryIndicator : Inport  Port=2
  From1 : From  Commented=on  GotoTag=DEMUpdation_Trigger  TagVisibility=global
  Manual Switch : ManualSwitch  CurrentSetting=0
  Mux : Mux  Commented=on  Inputs=2
  Scope : Scope
  Scope1 : Scope  Commented=on
  Unit Delay : UnitDelay  Commented=on  InitialCondition=InitialPlanningParameter  SampleTime=-1  HasFrameUpgradeWarning=on
  UpdateDEM : Subsystem  Commented=on
  Out1 : Outport  InitialOutput=[0 1 0 0 2 2 2 40 V*3.6]
  tag scope: Trajectory_Parameter=global
  wires:
  TrajectoryIndicator/1 -> UpdateDEM/2(TrajectoryIndicator)
  From1/1 -> Mux/1, UpdateDEM/Trigger
  ? -> Manual Switch/2
  Manual Switch/1 -> Scope/1, [Trajectory_Parameter], Out1/1
  UpdateDEM/1(PlanningParameter) -> Unit Delay/1
  Unit Delay/1 -> Manual Switch/1
  UpdateDEM/2(Expected_QueryID) -> Mux/2
  Mux/1 -> Scope1/1
  FeedBack/1 -> UpdateDEM/1(FeedBack_FromDriver)

== system Prescan_Carsim_0118_repair_cs/BMW_X5_SUV_1/Data Record Management ==
  Mux2 : Mux  Inputs=2
  Scope1 : Scope
  To File : ToFile  Filename=Parameter_TrajectoryIndicator.mat  SaveFormat=Timeseries
      settings: Decimation=40
  Vector Concatenate : Concatenate  NumInputs=3  Mode=Multidimensional array
  wires:
  Mux2/1 -> Scope1/1
  [Trajectory_Parameter] -> Vector Concatenate/1
  Vector Concatenate/1 -> To File/1
  [Curve_Flag] -> Mux2/1, Vector Concatenate/2
  [TrajectoryIndicator] -> Mux2/2, Vector Concatenate/3

== system Prescan_Carsim_0118_repair_cs/BMW_X5_SUV_1/DriverFeedBack ==
  note: Note: The value of these two constant block was assigned by the real drivers from the GUI
  note: Real Drivers
  note: Simulated Driver
  TrajectoryIndicator : Inport
  DEMUpdate_TriggerSignal : Constant
      settings: AttributesFormatString=|
      | Toggle within (0,1), each toggle trigger
      | the DEM updation
  Data Type Conversion : DataTypeConversion  Commented=on  OutDataTypeStr=double
  Demux : Demux  Outputs=2
  FeedBackFromDriver : Constant  Value=2
  From1 : From  Commented=on  GotoTag=Curve_Flag  TagVisibility=global
  From2 : From  Commented=on  GotoTag=Curve_Flag  TagVisibility=global
  Generate the FeedBack Obtainment Trigger Signal : Subsystem  Commented=on
  Mux : Mux  Commented=on  Inputs=2
  Mux1 : Mux  Inputs=2
  Mux2 : Mux  Commented=on
  Real-Simulattion-Driver-Switch : Constant  Value=0
      settings: AttributesFormatString=The value was assined by the GUI
  Scope2 : Scope  Commented=on
  Switch : Switch  Criteria=u2 > Threshold  Threshold=0.5
  driver evaluation model : Subsystem  Commented=on
  FeedBack : Outport
  tag scope: DEMUpdation_Trigger=global
  wires:
  Generate the FeedBack Obtainment Trigger Signal/1(Trigger Signal of Feedback obtainement) -> driver evaluation model/Trigger, Data Type Conversion/1
  DEMUpdate_TriggerSignal/1 -> Mux1/2
  driver evaluation model/2(FeedBack_Trigger) -> Mux/2, Mux2/4
  From1/1 -> Generate the FeedBack Obtainment Trigger Signal/1(CurveFlag)
  Demux/1 -> FeedBack/1
  Data Type Conversion/1 -> Mux2/2
  TrajectoryIndicator/1 -> driver evaluation model/1(TrajectoryIndicators)
  Mux2/1 -> Scope2/1
  From2/1 -> Mux2/1
  driver evaluation model/1(feedback) -> Mux/1, Mux2/3
  FeedBackFromDriver/1 -> Mux1/1
  Mux/1 -> Switch/1
  Mux1/1 -> Switch/3
  Real-Simulattion-Driver-Switch/1 -> Switch/2
  Switch/1 -> Demux/1
  Demux/2 -> [DEMUpdation_Trigger]

== system Prescan_Carsim_0118_repair_cs/BMW_X5_SUV_1/Dynamics_Empty ==
  note: For state mode 'Dynamic' positions
      | are not taken into account, as they
      | are computed by integrating velocity.
      | Click annotation for Help.
  MuxState : Subsystem  Tag=mux/State  mask(Empty Dynamics State Block){positioningmode=on, TimeStep=1/1000}
      mask prompts: positioningmode "Positioning Mode"; TimeStep "Auto Assigned: Time Step [s]"
      mask help:
      | Build the state of an actor based on user input.
      | The user can either use positioning mode or dynamics mode.
      | - When using positioning mode the position and orientation of the actor are set directly based on the input. Expected input is relative to the initial position and orientation of the actor. It's also possible to specify the velocity of the actor, though this input isn't used, only passed on.
      | - When using dynamics mode the position input is ignored. Expected input is velocity and orientation. The velocity is relative the current orientation of the actor, while orientation is relative to its initial orientation. The position of the actor is calculated based on the velocity and orientation given.
      settings: DeleteFcn=PreScanBlockDeleteFcn;
  STATE_BMW_X5_SUV_1 : Subsystem  Tag=mux/StatePort  Priority=0  LoadFcn=load PrescanStateActuatorData  mask(PreScan Sink Block: State){x0=Prescan_Carsim_1230_cs_be02757d7f212dd5, y0=Prescan_Carsim_1230_cs_6cfd759b89b9fc85, z0=Prescan_Carsim_1230_cs_08c5eb9a1bd7376a, Roll0=Prescan_Carsim_1230_cs_ac716d34d49f74ab, Pitch0=Prescan_Carsim_1230_cs_9435cc1cceb5050d, Yaw0=Prescan_Carsim_1230_cs_0658e9ca1334a8be, TimeStep=1/1000}
      mask prompts: x0 "Ini x-position VEHICLE wrt GLOBAL axis system [m]"; y0 "Ini y-position VEHICLE wrt GLOBAL axis system [m]"; z0 "Ini z-position VEHICLE wrt GLOBAL axis system [m]"; Roll0 "Ini roll-angle BODY wrt VEHICLE axis system [deg]"; Pitch0 "Ini pitch-angle BODY wrt VEHICLE axis system [deg]"; Yaw0 "Ini yaw-angle VEHICLE wrt GLOBAL axis system [deg]"; TimeStep "Auto-Assigned: Upload Period [s]"
      mask help:
      | The Actor State contains a vector signal of size (9x1), containing the following signals:
      |
      | -  Position                  (x,y,z)                                     [m]
      | -  Velocity                  (vx,vy,vz)                               [m/s]
      | -  Angles                    (Roll, Pitch, Yaw)                   [rad]
      |
      | The Actor state is defined in the global axis system.
      | The state is superponed on the Initial position defined in the GUI.
      |
      | For more information, please click Help.
      settings: DeleteFcn=PreScanBlockDeleteFcn;
      mask Help: eval('openHelp(222)')
      mask Display: image(imread('State.png'))
  State : Outport  Tag=outport/StateOutport  SampleTime=1/1000
  wires:
  MuxState/1(state) -> STATE_BMW_X5_SUV_1/1(State)
  STATE_BMW_X5_SUV_1/1(StateBus) -> State/1

== system Prescan_Carsim_0118_repair_cs/BMW_X5_SUV_1/JointGroup_WheelDisplacement_V2R ==
  Velocity [m/s] : Inport  SampleTime=TimeStep
  Discrete-Time Integrator : DiscreteIntegrator  SampleTime=TimeStep  ICPrevOutput=DiscIntNeverNeededParam  ICPrevScaledInput=DiscIntNeverNeededParam
  omega=V/Rwheel : Gain  Gain=1/TireRadius
  Rotation [rad] : Outport
  wires:
  Discrete-Time Integrator/1 -> Rotation [rad]/1  "roty"
  omega=V/Rwheel/1 -> Discrete-Time Integrator/1  "rotational speed [rad/s]"
  Velocity [m/s]/1 -> omega=V/Rwheel/1
